simulink model "ecssimulink"  (R2015b)
settings: Solver=FixedStepAuto  StartTime=0.0  StopTime=1  FixedStep=0.001  RelTol=1e-3
values from neighbouring files (symbols this model uses):
  A = [-2*(Caf + Car)/(mv*vx), -1-2*(lf * Caf - lr * Car)/(mv*vx*vx); -2*(lf * Caf - lr * Car)/Iz , -2*(lf*lf*Caf + lr*lr*Car)/(Iz*vx)]    [ecs.m]    (also in ssmodel.m = [ 0 1; 0 0 ]; ssmodel2.m = [0 1 0; 0 0 -rw/Iw; 0 0 0])
  beta_max = 0.4    [ecs.m]
  Bu = [0 ; 1/Iz]    [ecs.m]
  G = [2*Caf/(mv * vx) 2*lf*Caf/(Iz)]    [ecs.m]    (also in ssmodel2.m = [5 ; 10])
  gamma = sys_bicycle_dis.b(:,1)    [ecs.m]
  gamma_aug = [0;gamma]    [ecs.m]
  H = [0 1]    [ecs.m]
  Kus = 10    [ecs.m]
  lf = 1.141    [ecs.m]
  lr = 1.639    [ecs.m]
  Mz_max = 2    [ecs.m]
  phi = sys_bicycle_dis.a    [ecs.m]
  phi_aug = [1, H; [0;0], phi]    [ecs.m]
  r_max = 1    [ecs.m]
  rho = 1    [ecs.m]
settings Model: Creator=ADMIN  LastModifiedBy=ADMIN

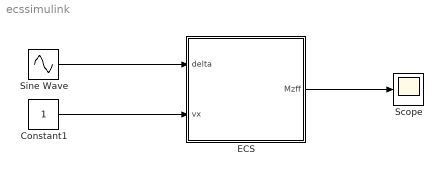
== system ecssimulink ==
  Constant1 : Constant
  ECS : MATLAB Function  InitFcn=|  TreatAsAtomicUnit=on
      | clc
      | clear all
      | 
      | Caf = 0.5;
      | Car = 0.3;
      | lf = 1.35;
      | lr = 1.23;
      | mv = 1529.98;
      | vx = 0.5;
      | Iz = 4605;
      | Kus = 10;
      | delta = 0.2;
      | rho = 1;
      | beta_max = 0.4;
      | r_max = 1;
      | Mz_max = 2;
      | 
      | A = [-2*(Caf + Car)/(mv*vx), -1-2*(lf * Caf - lr * Car)/(mv*vx*vx); -2*(lf * Caf - lr * Car)/Iz , -2*(lf*lf*Caf + lr*lr*Car)/(Iz*vx)];
      | Bu = [0 ; 1/Iz];
      | Bu_aug = [0, 2*Caf/(mv * vx); 1/Iz, 2*lf*Caf/(Iz)];
      | G = [2*Caf/(mv * vx) 2*lf*Caf/(Iz)];
      | 
      | sys_bicycle = ss(A,Bu_aug,[0 0],[0 0]);
      | sys_bicycle_dis = c2d(sys_bicycle, 0.001);
      | 
      | phi = sys_bicycle_dis.a;
      | gamma = sys_bicycle_dis.b(:,1);
      | H = [0 1];
      | 
      | phi_aug = [1, H; [0;0], phi];
      | gamma_aug = [0;gamma];
      | gamma_r = [1; 0 ; 0];
  Scope : Scope
  Sine Wave : Sin  Amplitude=0.1  Bias=0.5  SampleTime=0
  wires:
  Constant1/1 -> ECS/2(vx)
  ECS/1(Mzff) -> Scope/1
  Sine Wave/1 -> ECS/1(delta)

== matlab function ecssimulink/ECS ==
  data: delta input; vx input; Kus parameter; beta_max parameter; r_max parameter; Mz_max parameter; rho parameter; lf parameter; lr parameter; phi_aug parameter; gamma_aug parameter; phi parameter; gamma parameter; H parameter; Mzff output; A parameter; Bu parameter; G parameter
function Mzff  = fcn(delta, vx, Kus, beta_max, r_max, Mz_max, rho, lf, lr, phi_aug, gamma_aug, phi, gamma, H, A,Bu,G)
%#codegen

rd = vx / ((lf+lr) + Kus * vx *vx) * delta;

Q = diag([rho, 1/(beta_max * beta_max), 1/(r_max * r_max)]);
R = 1 / (Mz_max * Mz_max);

coder.extrinsic('dare');
P = eye(3);
P = dare(phi_aug, gamma_aug, Q, R);
Ka = inv(gamma_aug' * P * gamma_aug + R)*(gamma_aug'*P*phi_aug)

K = Ka(2:3);
Ki = Ka(1);

N_aug = inv([phi - eye(2), gamma; H, 0])*[0;0;1]
Nx = N_aug(1:2);
Nu = N_aug(3);
N_bar = Nu + K * Nx
Mzff = (G(1)*A(2,2)-G(2)*A(1,2))/(A(1,2)*Bu(2)) * delta
